simulink model "Opt_Tanque02"  (R2013a)
settings: Solver=ode45  StartTime=0.0  StopTime=400  RelTol=1e-3
InitFcn:
  | load('Kpm.mat')
  | load('Kdm.mat')
  | load('Kim.mat')
undefined symbols (not defined in the file or in its folder): sigbuilder_block
undefined symbols (not defined in the file): Kdm, Kim, Kpm
settings Model: Creator=Cristhian Ivan  LastModifiedBy=Cristhian Ivan

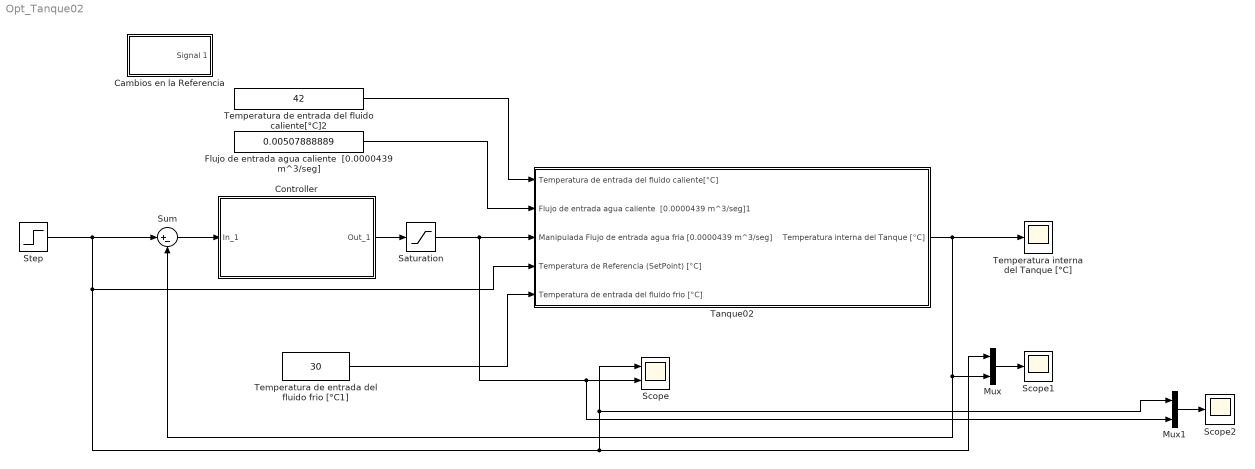
== system Opt_Tanque02 ==
  "Cambios en la Referencia " : Subsystem  Tag=STV Subsys  LoadFcn=sigbuilder_block('load');  StartFcn=sigbuilder_block('start');  StopFcn=sigbuilder_block('stop');  ClipboardFcn=sigbuilder_block('clipboard');  mask(Sigbuilder block){}
      mask help: Simulink:masks:SigbuilderBlock_MD
      mask init:
      | if ~strcmp(get_param(bdroot(gcbh),'SimulationStatus'),'stopped') tuvar = sigbuilder_block('maskInit'); end
      settings: CopyFcn=sigbuilder_block('copy');  DeleteFcn=sigbuilder_block('delete');  ModelCloseFcn=sigbuilder_block('modelClose');  PreSaveFcn=sigbuilder_block('preSave');  PauseFcn=sigbuilder_block('pause');  ContinueFcn=sigbuilder_block('continue');  NameChangeFcn=sigbuilder_block('namechange');  OpenFcn=sigbuilder_block('open',[437.25 118.5 550.5 394.5 ]);  CloseFcn=sigbuilder_block('close');
      mask Display: plot(0, 0, 100, 100,[2, 2, 32, 32, 2], [68, 8, 8, 68, 68],[32, 2], [38, 38], [32, 19, 2],[53, 60, 44], [32, 17, 17, 2],[16, 16, 31, 31]);txt = getActiveGroup(gcbh);text(2, 100, txt,'verticalAlignment', 'top');
  Controller : Subsystem  mask(PID Controller){P=Kpm, I=Kim, D=Kdm}
      mask prompts: P "Proportional:"; I "Integral"; D "Derivative:"
      mask help: Enter expressions for proportional, integral, and derivative terms.
      mask Help: This block implements a PID controller where paramaters are entered for the Proportional, Integral and Derivative terms.
      mask Display: disp('PID')
  "Flujo de entrada agua caliente  [0.0000439 m^3/seg] " : Constant  Value=0.00507888889
  Mux : Mux  Inputs=2
  Mux1 : Mux  Inputs=2
  Saturation : Saturate  UpperLimit=100  LowerLimit=0  ZeroCross=off
  Scope : Scope  NumInputPorts=2
      settings: YMin=-5~-5  YMax=5~5
  Scope1 : Scope
      settings: SaveName=ScopeData2
  Scope2 : Scope
      settings: SaveName=ScopeData3
  Step : Step  Time=0  After=38  SampleTime=0
  Sum : Sum  Inputs=|+-
  Tanque02 : Subsystem
  Temperatura de entrada del fluido caliente[°C]2 : Constant  Value=42
  Temperatura de entrada del fluido frio [°C1] : Constant  Value=30
  Temperatura interna del Tanque [°C] : Scope
      settings: TimeRange=10  YMin=20  YMax=45  SaveName=TransResp
  wires:
  Temperatura de entrada del fluido frio [°C1]/1 -> Tanque02/5(Temperatura de entrada del fluido frio [°C])
  Temperatura de entrada del fluido caliente[°C]2/1 -> Tanque02/1(Temperatura de entrada del fluido caliente[°C])
  "Flujo de entrada agua caliente  [0.0000439 m^3/seg] "/1 -> Tanque02/2(Flujo de entrada agua caliente  [0.0000439 m^3/seg]1)
  Controller/1(Out_1) -> Saturation/1
  Sum/1 -> Controller/1(In_1)
  Step/1 -> Scope/1, Mux1/1, Mux/1, Tanque02/4(Temperatura de Referencia (SetPoint) [°C]), Sum/1
  Tanque02/1(Temperatura interna del Tanque [°C]) -> Temperatura interna del Tanque [°C]/1, Sum/2, Mux/2
  Mux/1 -> Scope1/1
  Saturation/1 -> Mux1/2, Scope/2, Tanque02/3(Manipulada Flujo de entrada agua fria [0.0000439 m^3/seg])
  Mux1/1 -> Scope2/1

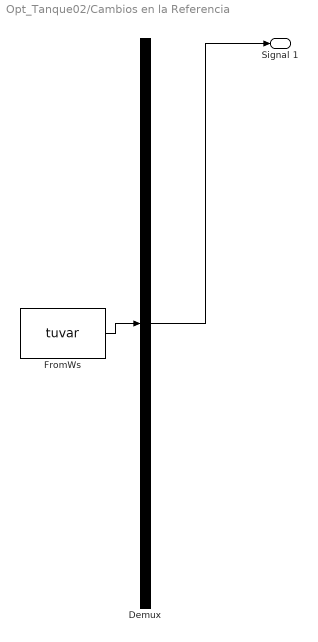
== system Opt_Tanque02/Cambios en la Referencia  ==
  Demux : Demux  Tag=STV Demux  Outputs=1
  FromWs : FromWorkspace  Tag=STV FromWs  VariableName=tuvar  SampleTime=0
      SigBuilderData=|
      | common.afterFinalStr = 'Extrapolate'
      | common.sampleTime = 0
      | dataSet.timeRange = [0 400]
      | dataSet.name = 'Group 1'
      | sbobj.Groups.Name = 'Group 1'
      | sbobj.Groups.Signals.Name = 'Signal 1'
      | sbobj.Groups.Signals.XData = [0 32 32 150 150 300 300 357 357 400]
      | sbobj.Groups.Signals.YData = [33 33 35.95 35.95 35 35 38.05 38.05 33.4 33.4]
      | sbobj.Groups.TimeRange = [0 400]
  Signal 1 : Outport  Tag=STV Outport
  wires:
  Demux/1 -> Signal 1/1
  FromWs/1 -> Demux/1

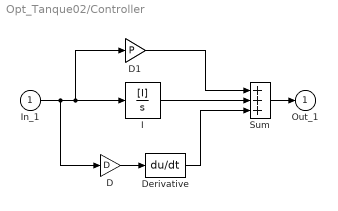
== system Opt_Tanque02/Controller ==
  In_1 : Inport
  D : Gain  Gain=D  SaturateOnIntegerOverflow=on  OutDataTypeStr=Inherit: Same as input  ParamDataTypeStr=Inherit: Same as input
  D1 : Gain  Gain=P  SaturateOnIntegerOverflow=on  OutDataTypeStr=Inherit: Same as input  ParamDataTypeStr=Inherit: Same as input
  Derivative : Derivative
  I : TransferFcn  Numerator=[I]  Denominator=[1 0]
  Sum : Sum  Inputs=+++  SaturateOnIntegerOverflow=on  InputSameDT=on  OutDataTypeStr=Inherit: Same as first input
  Out_1 : Outport  InitialOutput=0
  wires:
  In_1/1 -> D1/1, I/1, D/1
  Sum/1 -> Out_1/1
  D/1 -> Derivative/1
  Derivative/1 -> Sum/3
  I/1 -> Sum/2
  D1/1 -> Sum/1

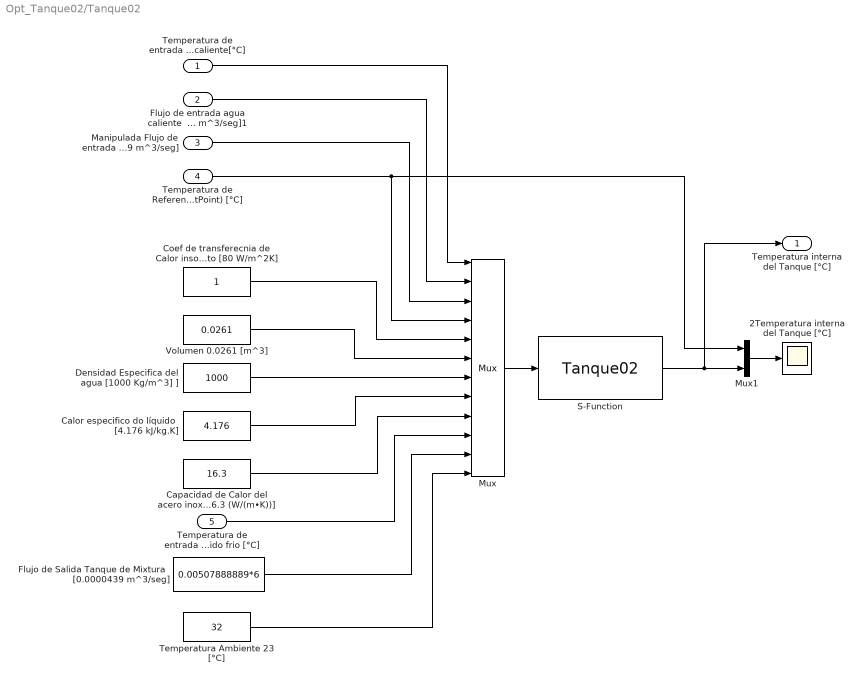
== system Opt_Tanque02/Tanque02 ==
  Temperatura de entrada del fluido caliente[°C] : Inport
  Flujo de entrada agua caliente  [0.0000439 m^3/seg]1 : Inport  Port=2
  Manipulada Flujo de entrada agua fria [0.0000439 m^3/seg] : Inport  Port=3
  Temperatura de Referencia (SetPoint) [°C] : Inport  Port=4
  Temperatura de entrada del fluido frio [°C] : Inport  Port=5
  2Temperatura interna del Tanque [°C] : Scope
      settings: TimeRange=10  YMin=34.9625  YMax=35
  Calor especifico do líquido  [4.176 kJ/kg.K] : Constant  Value=4.176
  Capacidad de Calor del acero inox [16.3 (W/(m•K))] : Constant  Value=16.3
  Coef de transferecnia de Calor insolamiento [80 W/m^2K] : Constant
  Densidad Especifica del agua [1000 Kg/m^3] ] : Constant  Value=1000
  Flujo de Salida Tanque de Mixtura  [0.0000439 m^3/seg] : Constant  Value=0.00507888889*6
  Mux : Mux  Inputs=12
  Mux1 : Mux  Inputs=2
  S-Function : S-Function  FunctionName=Tanque02  EnableBusSupport=off
  "Temperatura Ambiente 23 [°C] " : Constant  Value=32
  Volumen 0.0261 [m^3] : Constant  Value=0.0261
  Temperatura interna del Tanque [°C] : Outport
  wires:
  Temperatura de entrada del fluido frio [°C]/1 -> Mux/10
  Volumen 0.0261 [m^3]/1 -> Mux/6
  Capacidad de Calor del acero inox [16.3 (W/(m•K))]/1 -> Mux/9
  Calor especifico do líquido  [4.176 kJ/kg.K]/1 -> Mux/8
  S-Function/1 -> Temperatura interna del Tanque [°C]/1, Mux1/2
  Coef de transferecnia de Calor insolamiento [80 W/m^2K]/1 -> Mux/5
  Mux/1 -> S-Function/1
  Densidad Especifica del agua [1000 Kg/m^3] ]/1 -> Mux/7
  Flujo de Salida Tanque de Mixtura  [0.0000439 m^3/seg]/1 -> Mux/11
  "Temperatura Ambiente 23 [°C] "/1 -> Mux/12
  Mux1/1 -> 2Temperatura interna del Tanque [°C]/1
  Temperatura de entrada del fluido caliente[°C]/1 -> Mux/1
  Manipulada Flujo de entrada agua fria [0.0000439 m^3/seg]/1 -> Mux/3
  Flujo de entrada agua caliente  [0.0000439 m^3/seg]1/1 -> Mux/2
  Temperatura de Referencia (SetPoint) [°C]/1 -> Mux1/1, Mux/4
